simulink model "heat_exchanger_PID_Valve"  (R2018a)
settings: Solver=VariableStepAuto  StartTime=0.0  StopTime=1000  RelTol=1e-3
values from neighbouring files (symbols this model uses):
  Area = n*A_heat_plate    (= 9.8716)    [heat_exchanger_config.m]    (also in linearization.m = 20)
  cp_H2O = 4190    [heat_exchanger_config.m]    (also in linearization.m)
  cp_wort = 4062    [heat_exchanger_config.m]    (also in linearization.m = 4000)
  HE_delay = 15    [heat_exchanger_config.m]    (also in linearization.m = 5)
  m_H2O = m_wort    (= 10)    [heat_exchanger_config.m]    (also in linearization.m = 1)
  m_wort = 10    [heat_exchanger_config.m]    (also in linearization.m = 1)
  rho_wort = 1.06    [heat_exchanger_config.m]    (also in linearization.m)
  T_H2O_in = 5    [heat_exchanger_config.m]    (also in linearization.m = 10)
  T_wort_in = 95    [heat_exchanger_config.m]    (also in linearization.m = 70)
  U = (m_dot_h_data*cp_wort*(T_wort_in-T_wort_out)*log(Delta_T2/Delta_T1))/     (Area*(Delta_T2-Delta_T1))    [heat_exchanger_config.m]    (also in linearization.m = 1000)
libraries: elec_lib x6, simulink x3, fl_lib x3, nesl_utility x3
settings Model: Creator=Alexander  LastModifiedBy=Oscar
settings SolverCC: ZeroCrossAlgorithm=Adaptive
settings DebuggingCC: MaxConsecutiveZCsMsg=none

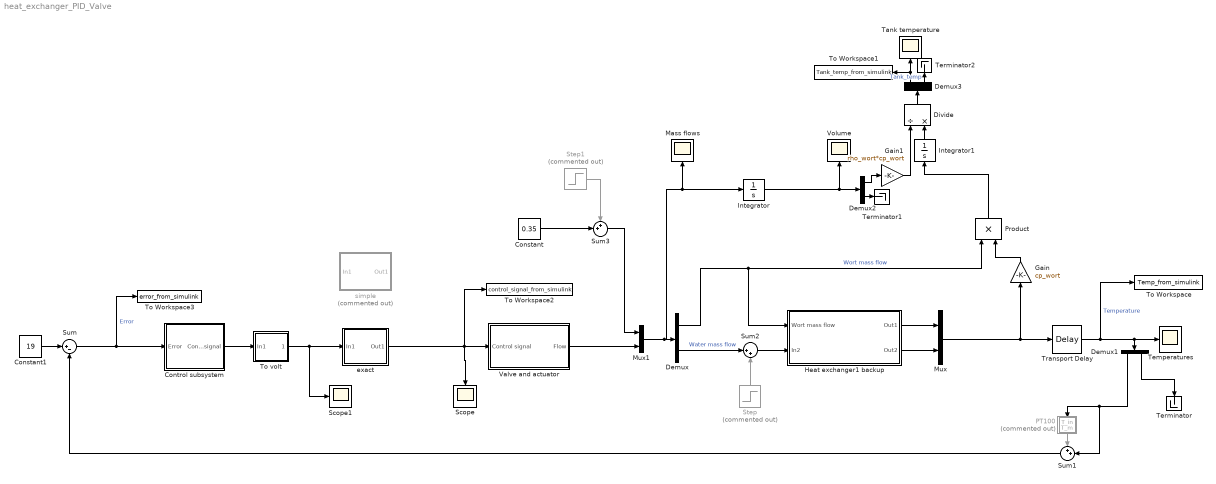
== system heat_exchanger_PID_Valve ==
  Constant : Constant  Value=0.35
  Constant1 : Constant  Value=19
  "Control subsystem " : Subsystem
  Demux{,1..3} (4 alike) : Demux  Outputs=2
  Divide : Product  Inputs=/*
  Gain : Gain  Gain=cp_wort
  Gain1 : Gain  Gain=rho_wort*cp_wort
  Heat exchanger1 backup : Subsystem
  Integrator : Integrator
  Integrator1 : Integrator
  Mass flows : Scope
  Mux : Mux  Inputs=2
  Mux1 : Mux  Inputs=2
  PT100 : Subsystem  Commented=on
  Product : Product
  Scope : Scope
  Scope1 : Scope
  Step : Step  Commented=on  Time=500  After=-0.1  SampleTime=0
  Step1 : Step  Commented=on  Time=500  After=0.105  SampleTime=0
  Sum : Sum  Inputs=|+-
  Sum1 : Sum  Inputs=++|
  Sum2 : Sum  Inputs=|++
  Sum3 : Sum  Inputs=++|
  Tank temperature : Scope
  Temperatures : Scope
  Terminator : Terminator
  Terminator1 : Terminator
  Terminator2 : Terminator
  To Workspace : ToWorkspace  VariableName=Temp_from_simulink  SaveFormat=Timeseries  SampleTime=-1
  To Workspace1 : ToWorkspace  VariableName=Tank_temp_from_simulink  SaveFormat=Timeseries  SampleTime=-1
  To Workspace2 : ToWorkspace  VariableName=control_signal_from_simulink  SaveFormat=Timeseries  SampleTime=-1
  To Workspace3 : ToWorkspace  VariableName=error_from_simulink  SaveFormat=Timeseries  SampleTime=-1
  To volt : Subsystem
  Transport Delay : TransportDelay  DelayTime=HE_delay
  Valve and actuator : Subsystem
  Volume : Scope
  exact : Subsystem
  simple : Subsystem  Commented=on
  wires:
  Demux/1 -> Product/1, Heat exchanger1 backup/1(Wort mass flow)  "Wort mass flow"
  Mux/1 -> Transport Delay/1, Gain/1
  Integrator/1 -> Demux2/1, Volume/1
  Transport Delay/1 -> Temperatures/1, Demux1/1, To Workspace/1  "Temperature"
  Mux1/1 -> Demux/1, Integrator/1, Mass flows/1
  Demux1/1 -> PT100/1(T_in), Sum1/2
  Constant1/1 -> Sum/1
  Integrator1/1 -> Divide/2
  Gain1/1 -> Divide/1
  Product/1 -> Integrator1/1
  Gain/1 -> Product/2
  Demux2/1 -> Gain1/1
  Demux2/2 -> Terminator1/1
  Demux3/2 -> Terminator2/1
  Divide/1 -> Demux3/1
  Demux3/1 -> Tank temperature/1, To Workspace1/1  "Tank_temp"
  Sum/1 -> "Control subsystem "/1(Error), To Workspace3/1  "Error"
  PT100/1(T_m) -> Sum1/1
  Sum1/1 -> Sum/2
  Demux/2 -> Sum2/1  "Water mass flow"
  Step/1 -> Sum2/2
  Demux1/2 -> Terminator/1
  Valve and actuator/1(Flow) -> Mux1/2
  Sum2/1 -> Heat exchanger1 backup/2(In2)
  Heat exchanger1 backup/1(Out1) -> Mux/1
  Heat exchanger1 backup/2(Out2) -> Mux/2
  To volt/1(Out1) -> exact/1(In1), Scope1/1
  "Control subsystem "/1(Control signal) -> To volt/1(In1)
  Sum3/1 -> Mux1/1
  Constant/1 -> Sum3/2
  Step1/1 -> Sum3/1
  exact/1(Out1) -> Scope/1, To Workspace2/1, Valve and actuator/1(Control signal)

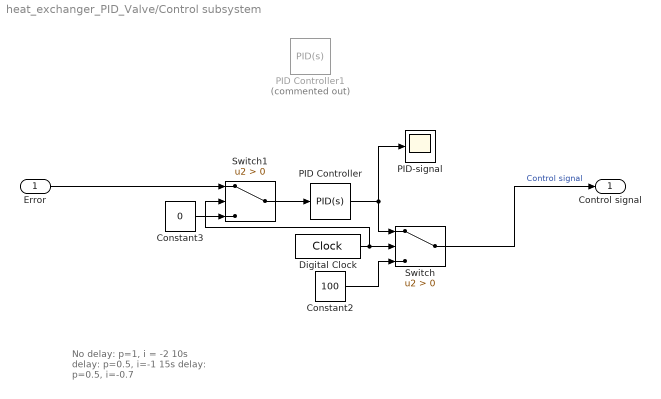
== system heat_exchanger_PID_Valve/Control subsystem  ==
  note: No delay: p=1, i = -2
      | 10s delay: p=0.5, i=-1
      | 15s delay: p=0.5, i=-0.7
  Error : Inport
  Constant2 : Constant  Value=100
  Constant3 : Constant  Value=0
  Digital Clock : DigitalClock
  PID Controller : simulink/Continuous/PID Controller  Controller=PID  TimeDomain=Continuous-time  SampleTime=-1  IntegratorMethod=Forward Euler  FilterMethod=Forward Euler  Form=Parallel  UseFilter=on  ControllerParametersSource=internal  P=3  I=-0.8  D=1  N=100  InitialConditionSource=internal  InitialConditionForIntegrator=0  InitialConditionForFilter=0  ExternalReset=none  LimitOutput=on  UpperSaturationLimit=850  LowerSaturationLimit=0  LinearizeAsGain=on  AntiWindupMode=back-calculation  Kb=1  TrackingMode=off  Kt=1  PParamMin=[]  PParamMax=[]  IParamMin=[]  IParamMax=[]  DParamMin=[]  DParamMax=[]  NParamMin=[]  NParamMax=[]  KbParamMin=[]  KbParamMax=[]  KtParamMin=[]  KtParamMax=[]  POutMin=[]  POutMax=[]  IOutMin=[]  IOutMax=[]  DOutMin=[]  DOutMax=[]  NOutMin=[]  NOutMax=[]  KbOutMin=[]  KbOutMax=[]  KtOutMin=[]  KtOutMax=[]  IntegratorOutMin=[]  IntegratorOutMax=[]  FilterOutMin=[]  FilterOutMax=[]  SumOutMin=[]  SumOutMax=[]  SumI1OutMin=[]  SumI1OutMax=[]  SumI2OutMin=[]  SumI2OutMax=[]  SumI3OutMin=[]  SumI3OutMax=[]  SumDOutMin=[]  SumDOutMax=[]  SaturationOutMin=[]  SaturationOutMax=[]  IntegratorContinuousStateAttributes=''  IntegratorStateMustResolveToSignalObject=off  IntegratorRTWStateStorageClass=Auto  FilterContinuousStateAttributes=''  FilterStateMustResolveToSignalObject=off  FilterRTWStateStorageClass=Auto  DifferentiatorICPrevScaledInput=0  DifferentiatorOutMin=[]  DifferentiatorOutMax=[]  InitialConditionSetting=State (most efficient)  FilterDiffOutCoefMin=[]  FilterDiffOutCoefMax=[]  SumDenOutMin=[]  SumDenOutMax=[]  SumNumOutMin=[]  SumNumOutMax=[]  ReciprocalOutMin=[]  ReciprocalOutMax=[]  DivideOutMin=[]  DivideOutMax=[]  TunerSelectOption=Transfer Function Based (PID Tuner App)
  PID Controller1 : simulink/Continuous/PID Controller  Commented=on  Controller=PID  TimeDomain=Continuous-time  SampleTime=-1  IntegratorMethod=Forward Euler  FilterMethod=Forward Euler  Form=Parallel  UseFilter=on  ControllerParametersSource=internal  P=1  I=-2  D=0  N=100  InitialConditionSource=internal  InitialConditionForIntegrator=0  InitialConditionForFilter=0  ExternalReset=none  LimitOutput=on  UpperSaturationLimit=850  LowerSaturationLimit=0  LinearizeAsGain=on  AntiWindupMode=back-calculation  Kb=1  TrackingMode=off  Kt=1  PParamMin=[]  PParamMax=[]  IParamMin=[]  IParamMax=[]  DParamMin=[]  DParamMax=[]  NParamMin=[]  NParamMax=[]  KbParamMin=[]  KbParamMax=[]  KtParamMin=[]  KtParamMax=[]  POutMin=[]  POutMax=[]  IOutMin=[]  IOutMax=[]  DOutMin=[]  DOutMax=[]  NOutMin=[]  NOutMax=[]  KbOutMin=[]  KbOutMax=[]  KtOutMin=[]  KtOutMax=[]  IntegratorOutMin=[]  IntegratorOutMax=[]  FilterOutMin=[]  FilterOutMax=[]  SumOutMin=[]  SumOutMax=[]  SumI1OutMin=[]  SumI1OutMax=[]  SumI2OutMin=[]  SumI2OutMax=[]  SumI3OutMin=[]  SumI3OutMax=[]  SumDOutMin=[]  SumDOutMax=[]  SaturationOutMin=[]  SaturationOutMax=[]  IntegratorContinuousStateAttributes=''  IntegratorStateMustResolveToSignalObject=off  IntegratorRTWStateStorageClass=Auto  FilterContinuousStateAttributes=''  FilterStateMustResolveToSignalObject=off  FilterRTWStateStorageClass=Auto  DifferentiatorICPrevScaledInput=0  DifferentiatorOutMin=[]  DifferentiatorOutMax=[]  InitialConditionSetting=State (most efficient)  FilterDiffOutCoefMin=[]  FilterDiffOutCoefMax=[]  SumDenOutMin=[]  SumDenOutMax=[]  SumNumOutMin=[]  SumNumOutMax=[]  ReciprocalOutMin=[]  ReciprocalOutMax=[]  DivideOutMin=[]  DivideOutMax=[]  TunerSelectOption=Transfer Function Based (PID Tuner App)
  PID-signal : Scope
  Switch : Switch  Criteria=u2 > Threshold
  Switch1 : Switch  Criteria=u2 > Threshold
  Control signal : Outport
  wires:
  Constant3/1 -> Switch1/3
  Digital Clock/1 -> Switch1/2, Switch/2
  Switch1/1 -> PID Controller/1
  PID Controller/1 -> PID-signal/1, Switch/1
  Constant2/1 -> Switch/3
  Error/1 -> Switch1/1
  Switch/1 -> Control signal/1  "Control signal"

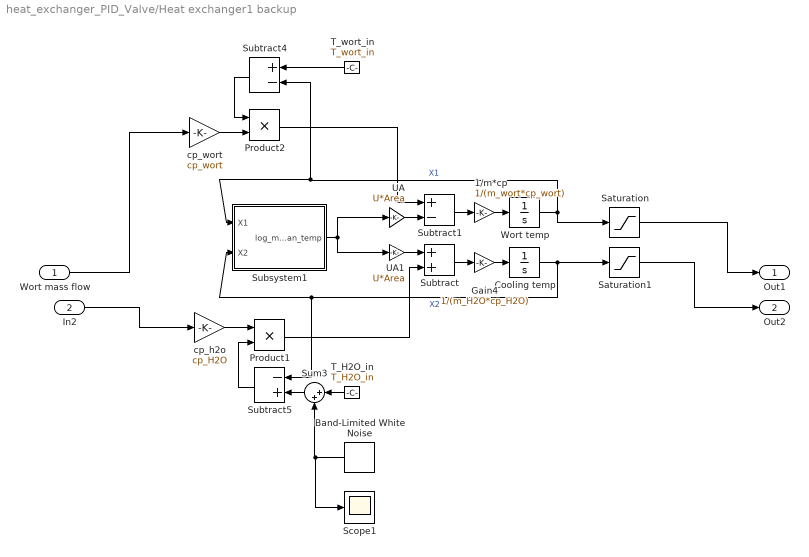
== system heat_exchanger_PID_Valve/Heat exchanger1 backup ==
  Wort mass flow : Inport
  In2 : Inport  Port=2
  "1/m*cp " : Gain  Gain=1/(m_wort*cp_wort)
  Band-Limited White Noise : simulink/Sources/Band-Limited White Noise  Cov=[5]  Ts=100  seed=[23341]
  Cooling temp : Integrator  InitialCondition=T_H2O_in-0.1
  Gain4 : Gain  Gain=1/(m_H2O*cp_H2O)
  Product1 : Product
  Product2 : Product
  Saturation : Saturate  UpperLimit=T_wort_in  LowerLimit=T_H2O_in
  Saturation1 : Saturate  UpperLimit=T_wort_in  LowerLimit=T_H2O_in
  Scope1 : Scope
  Subsystem1 : Subsystem
  Subtract : Sum
  Subtract1 : Sum  Inputs=+-
  Subtract4 : Sum  Inputs=+-
  Subtract5 : Sum  Inputs=-+
  Sum3 : Sum  Inputs=|++
  T_H2O_in : Constant  Value=T_H2O_in
  T_wort_in : Constant  Value=T_wort_in
  UA : Gain  Gain=U*Area
  "UA1 " : Gain  Gain=U*Area
  Wort temp : Integrator  InitialCondition=T_wort_in-0.1
  cp_h2o : Gain  Gain=cp_H2O
  cp_wort : Gain  Gain=cp_wort
  Out1 : Outport
  Out2 : Outport  Port=2
  wires:
  In2/1 -> cp_h2o/1
  cp_wort/1 -> Product2/2
  T_H2O_in/1 -> Sum3/1
  cp_h2o/1 -> Product1/1
  Saturation1/1 -> Out2/1
  Wort mass flow/1 -> cp_wort/1
  Subsystem1/1(log_mean_temp) -> UA/1, "UA1 "/1
  Subtract5/1 -> Product1/2
  Subtract4/1 -> Product2/1
  "1/m*cp "/1 -> Wort temp/1
  Wort temp/1 -> Saturation/1, Subsystem1/1("X1 "), Subtract4/2  "X1"
  Subtract/1 -> Gain4/1
  Sum3/1 -> Subtract5/2
  "UA1 "/1 -> Subtract/1
  Product2/1 -> Subtract1/1
  Saturation/1 -> Out1/1
  UA/1 -> Subtract1/2
  Cooling temp/1 -> Saturation1/1, Subtract5/1, Subsystem1/2(X2)  "X2"
  Band-Limited White Noise/1 -> Scope1/1, Sum3/2
  Gain4/1 -> Cooling temp/1
  T_wort_in/1 -> Subtract4/1
  Product1/1 -> Subtract/2
  Subtract1/1 -> "1/m*cp "/1

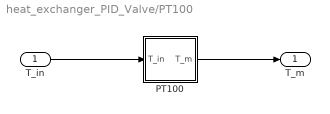
== system heat_exchanger_PID_Valve/PT100 ==
  T_in : Inport
  "PT100 " : MATLAB Function  TreatAsAtomicUnit=on
  T_m : Outport
  wires:
  T_in/1 -> "PT100 "/1(T_in)
  "PT100 "/1(T_m) -> T_m/1

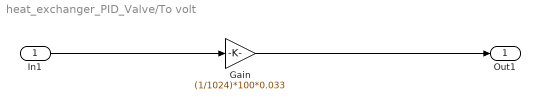
== system heat_exchanger_PID_Valve/To volt ==
  In1 : Inport
  Gain : Gain  Gain=(1/1024)*100*0.033
  Out1 : Outport
  wires:
  In1/1 -> Gain/1
  Gain/1 -> Out1/1

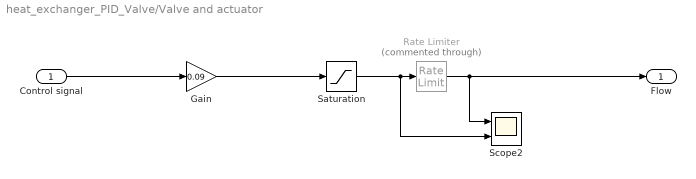
== system heat_exchanger_PID_Valve/Valve and actuator ==
  Control signal : Inport
  Gain : Gain  Gain=0.09
  Rate Limiter : RateLimiter  Commented=through  RisingSlewLimit=0.01  FallingSlewLimit=-0.01  SampleTimeMode=inherited
  Saturation : Saturate  UpperLimit=0.9  LowerLimit=0
  Scope2 : Scope  NumInputPorts=2
  Flow : Outport
  wires:
  Control signal/1 -> Gain/1
  Rate Limiter/1 -> Scope2/1, Flow/1
  Saturation/1 -> Scope2/2, Rate Limiter/1
  Gain/1 -> Saturation/1

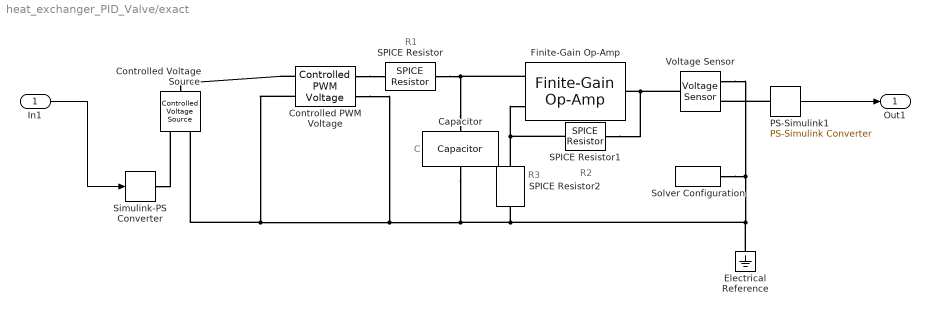
== system heat_exchanger_PID_Valve/exact ==
  note: C
  note: R2
  note: R1
  note: R3
  In1 : Inport
  Capacitor : elec_lib/Passive Devices/Capacitor  enable_table=0  c=10 uF  Cvec=[1e-05, 1e-06] F  Vvec=[0, 10] V  CV_table_symmetry=1  C_tol=5  enable_C_tol=0  tol_distribution=1  nSigma=4  r=1e-6 Ohm  g=0 1/Ohm  enable_operating_limits=0  operating_limit_action=2  max_working_voltage_range=[-25, 25] V  power_rating=1 W  enable_faults=0  fault_action=1  Cscale_faulted=100  R_faulted=1e-3 Ohm  G_faulted=0 1/Ohm  tau_fault=1e-3 s  enable_temporal_fault=0  t_fault=1 s  enable_behavioral_fault=0  max_permissible_voltage_range=[-100, 100] V  t_fail_on_voltage=1 s  i_specify=off  i_priority=None  i=0 A  i_nominal_specify=off  i_nominal_unit=A  i_nominal_value=1  v_specify=off  v_priority=None  v=0 V  v_nominal_specify=off  v_nominal_unit=V  v_nominal_value=1  vc_specify=off  vc_priority=High  vc=0 V  vc_nominal_specify=off  vc_nominal_unit=V  vc_nominal_value=1
  Controlled PWM Voltage : elec_lib/Actuators & Drivers/Drivers/Controlled PWM Voltage  F=1 kHz  TD=0 s  pulse_width_offset=0 s  pulse_min=0 s  Vmin=0 V  Vmax=5 V  Vm=3.3 V  pwm_or_av=1  event_type=1  sample_time=1e-6 s  u_min=0  u_max=1
      settings: SourceProductName=Simscape Electronics  SourceProductBaseCode=SN
  Controlled Voltage Source : fl_lib/Electrical/Electrical Sources/Controlled Voltage Source
  Electrical Reference : fl_lib/Electrical/Electrical Elements/Electrical Reference
  Finite-Gain Op-Amp : elec_lib/Integrated Circuits/Finite-Gain Op-Amp  A=1000  Rin=1e6 Ohm  Rout=100 Ohm  Vmin=-100 V  Vmax=100 V  noise_mode=0  v_noise=30e-9 V/Hz^0.50000  noise_prm=1  i_noise=0.5e-12 A/Hz^0.50000  ip_noise=0.5e-12 A/Hz^0.50000  in_noise=0.5e-12 A/Hz^0.50000  sample_time=1e-3 s  repeatability=1  auto_seed_v=3499211588  auto_seed_ip=3890346746  auto_seed_in=545404223  user_seed_v=0  user_seed_ip=0  user_seed_in=0
      settings: SourceProductName=Simscape Electronics  SourceProductBaseCode=SN
  PS-Simulink1 : nesl_utility/PS-Simulink Converter  PhysicalDomain=network_engine_domain  SubClassName=ps_output  LeftPortType=input  RightPortType=output  PseudoPeriodic=off  Frequencies=[]  Unit=V  AffineConversion=off
  SPICE Resistor : elec_lib/Additional Components/SPICE-Compatible Components/Passive Devices/SPICE Resistor  SCALE=1.0  R_param=1  R=1.3 kOhm  RSH=0 Ohm  LENGTH=1e-6 m  WIDTH=1e-6 m  NARROW=0 m  T_param=1  TC1=0 1/K  TC2=0 1/K^2  TOFFSET=0 K  TFIXED=300.15 K  TMEAS=300.15 K
      settings: SourceProductName=Simscape Electronics  SourceProductBaseCode=SN
  SPICE Resistor1 : elec_lib/Additional Components/SPICE-Compatible Components/Passive Devices/SPICE Resistor  SCALE=1.0  R_param=1  R=240 Ohm  RSH=0 Ohm  LENGTH=1e-6 m  WIDTH=1e-6 m  NARROW=0 m  T_param=1  TC1=0 1/K  TC2=0 1/K^2  TOFFSET=0 K  TFIXED=300.15 K  TMEAS=300.15 K
      settings: SourceProductName=Simscape Electronics  SourceProductBaseCode=SN
  SPICE Resistor2 : elec_lib/Additional Components/SPICE-Compatible Components/Passive Devices/SPICE Resistor  SCALE=1.0  R_param=1  R=118 Ohm  RSH=0 Ohm  LENGTH=1e-6 m  WIDTH=1e-6 m  NARROW=0 m  T_param=1  TC1=0 1/K  TC2=0 1/K^2  TOFFSET=0 K  TFIXED=300.15 K  TMEAS=300.15 K
      settings: SourceProductName=Simscape Electronics  SourceProductBaseCode=SN
  Simulink-PS Converter : nesl_utility/Simulink-PS Converter  PhysicalDomain=network_engine_domain  SubClassName=ps_input  LeftPortType=input  RightPortType=output  PseudoPeriodic=off  Frequencies=[]  NoiseDistribution=none  NoiseParameters=[]  Unit=1  AffineConversion=off  FilteringAndDerivatives=provide  SimscapeFilterOrder=1  InputFilterTimeConstant=0.001  UdotUserProvided=0
  Solver Configuration : nesl_utility/Solver Configuration  PhysicalDomain=network_engine_domain  SubClassName=solver  LeftPortType=input  RightPortType=generic  Tones=[]  Harmonics=[]  SimulateNoise=off  Profile=off  UseLocalSampling=off  EnableSwitchedLinearOptims=on  FrequencyDomain=off  UseCCode=off  RelTol=0.001  AbsTol=1e-06  MinStep=1e-09  ToWorkspace=off  RevertToSquareIcSolve=off  NumHomotopyIterations=100  PhasorMode=off  PhasorModeNumHarmonics=1  DoDC=off  ResidualTolerance=1e-9  UseLocalSolver=off  LocalSolverChoice=NE_BACKWARD_EULER_ADVANCER  LocalSolverSampleTime=.001  DoFixedCost=off  MaxNonlinIter=3  MaxModeIter=2  LinearAlgebra=Sparse  EquationFormulation=NE_TIME_EF  DelaysMemoryBudget=1024  AutomaticFiltering=on  FilteringTimeConstant=0.001
  Voltage Sensor : fl_lib/Electrical/Electrical Sensors/Voltage Sensor
  Out1 : Outport
  wires:
  PS-Simulink1/1 -> Out1/1
  In1/1 -> Simulink-PS Converter/1
  connections:
  Controlled PWM Voltage/LConn2 -- Voltage Sensor/RConn2 -- Solver Configuration/RConn1 -- Electrical Reference/LConn1 -- SPICE Resistor2/RConn1 -- Capacitor/RConn1 -- Controlled PWM Voltage/RConn2 -- Controlled Voltage Source/RConn2
  Finite-Gain Op-Amp/RConn1 -- SPICE Resistor1/LConn1 -- Voltage Sensor/LConn1
  Capacitor/LConn1 -- SPICE Resistor/RConn1 -- Finite-Gain Op-Amp/LConn1
  Finite-Gain Op-Amp/LConn2 -- SPICE Resistor2/LConn1 -- SPICE Resistor1/RConn1
  Controlled PWM Voltage/RConn1 -- SPICE Resistor/LConn1
  Simulink-PS Converter/RConn1 -- Controlled Voltage Source/RConn1
  Controlled PWM Voltage/LConn1 -- Controlled Voltage Source/LConn1
  PS-Simulink1/LConn1 -- Voltage Sensor/RConn1

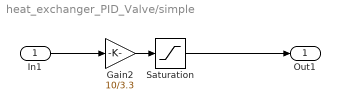
== system heat_exchanger_PID_Valve/simple ==
  In1 : Inport
  Gain2 : Gain  Gain=10/3.3
  Saturation : Saturate  UpperLimit=6.6  LowerLimit=0
  Out1 : Outport
  wires:
  Saturation/1 -> Out1/1
  In1/1 -> Gain2/1
  Gain2/1 -> Saturation/1

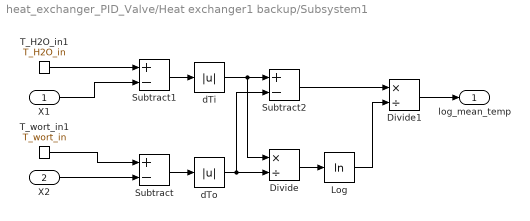
== system heat_exchanger_PID_Valve/Heat exchanger1 backup/Subsystem1 ==
  "X1 " : Inport
  X2 : Inport  Port=2
  Divide : Product  Inputs=*/
  Divide1 : Product  Inputs=*/
  Log : Math  Operator=log  SaturateOnIntegerOverflow=on
  Subtract : Sum  Inputs=+-
  Subtract1 : Sum  Inputs=+-
  Subtract2 : Sum  Inputs=+-
  T_H2O_in1 : Constant  Value=T_H2O_in
  T_wort_in1 : Constant  Value=T_wort_in
  dTi : Abs
  dTo : Abs
  log_mean_temp : Outport
  wires:
  Subtract/1 -> dTo/1
  T_wort_in1/1 -> Subtract/1
  X2/1 -> Subtract/2
  Subtract1/1 -> dTi/1
  "X1 "/1 -> Subtract1/2
  T_H2O_in1/1 -> Subtract1/1
  dTo/1 -> Subtract2/2, Divide/2
  dTi/1 -> Subtract2/1, Divide/1
  Divide/1 -> Log/1
  Log/1 -> Divide1/2
  Divide1/1 -> log_mean_temp/1
  Subtract2/1 -> Divide1/1

== matlab function heat_exchanger_PID_Valve/PT100/PT100  ==
  settings: updateMethod=DISCRETE
  data: T_in input; T_m output
function T_m = fcn(T_in)
%#codegen

%Sensor class
AA = 0.1;
A = 0.15;
B = 0.3;
C = 0.6;

aa = 0.0017;
a = 0.002;
b = 0.005;
c = 0.01;
% sensor = sensor_type;
% switch sensor
%     case 'AA'
%         T_m = randi([-1 1],1)*(rand(1)*AA + rand(1)*aa*T_in);
%     case 'A'
%         T_m = randi([-1 1],1)*(rand(1)*A + rand(1)*a*T_in);
%     case 'B'
%         T_m = randi([-1 1],1)*(rand(1)*B + rand(1)*b*T_in);
%     case 'C'
%         T_m = randi([-1 1],1)*(rand(1)*C + rand(1)*c*T_in);
% end



T_m = randi([-1 1],1)*(rand(1)*AA + rand(1)*aa*T_in);
